simulink model "Aufgabe4"  (R2022a)
settings: Solver=FixedStepAuto  StartTime=0.0  StopTime=10  FixedStep=0.01  RelTol=1e-3  EnableMultiTasking=on
settings Model: Creator=Simtp29  LastModifiedBy=yufu
settings SolverCC: AlgebraicLoopSolver=TrustRegion
settings DataIOCC: ReturnWorkspaceOutputs=off
settings DebuggingCC: UnconnectedInputMsg=warning  UnconnectedOutputMsg=warning  UnconnectedLineMsg=warning  SFMachineParentedDataDiag=warning  ArithmeticOperatorsInVariantConditions=warning
settings SFSimCC: SimUseLocalCustomCode=off  CustomCodeUndefinedFunction=UseInterfaceOnly
settings RTWCC: RTWUseLocalCustomCode=off

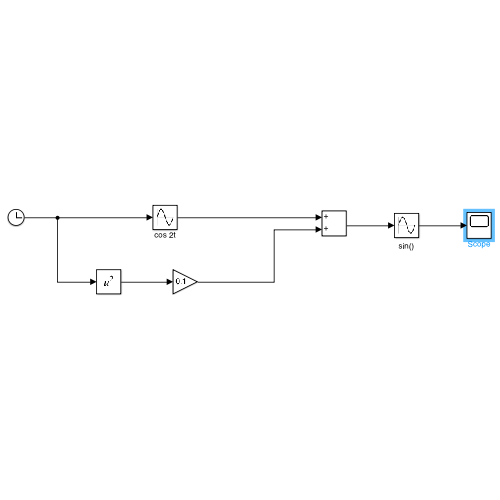
[thumbnail: Simulink's stored preview of the top-level diagram]
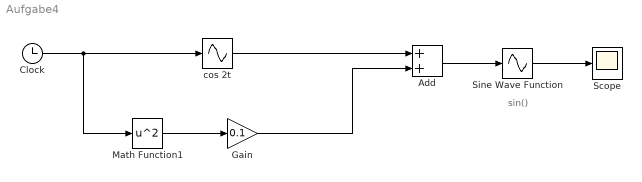
== system Aufgabe4 ==
  note: sin()
  Add : Sum
  Clock : Clock
  Gain : Gain  Gain=0.1
  Math Function1 : Math  Operator=square  SignedPower=on
  Scope : Scope
  Sine Wave Function : Sin  TimeSource=Use external signal  SampleTime=0
  "cos 2t " : Sin  TimeSource=Use external signal  Frequency=2  Phase=pi/2  SampleTime=0
  wires:
  Clock/1 -> Math Function1/1, "cos 2t "/1
  "cos 2t "/1 -> Add/1
  Add/1 -> Sine Wave Function/1
  Sine Wave Function/1 -> Scope/1
  Math Function1/1 -> Gain/1
  Gain/1 -> Add/2
